simulink model "test_control_lib_vect_sign_change"  (R2017a)
settings: Solver=VariableStepAuto  StartTime=0.0  StopTime=0.020*100  RelTol=1e-3
settings Model: Creator=CHIVFUR  LastModifiedBy=CHIVFUR

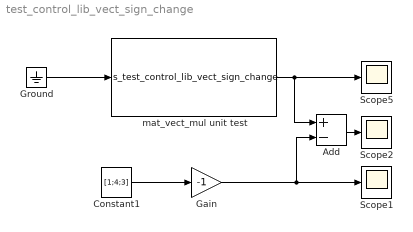
== system test_control_lib_vect_sign_change ==
  Add : Sum  Inputs=+-
  Constant1 : Constant  Value=[1;4;3]
  Gain : Gain  Gain=-1
  Ground : Ground
  Scope1 : Scope
  Scope2 : Scope
  Scope5 : Scope
  "mat_vect_mul unit test " : S-Function  FunctionName=s_test_control_lib_vect_sign_change  Parameters=1/30000  SFunctionDeploymentMode=off  EnableBusSupport=off
  wires:
  "mat_vect_mul unit test "/1 -> Scope5/1, Add/1
  Ground/1 -> "mat_vect_mul unit test "/1
  Constant1/1 -> Gain/1
  Add/1 -> Scope2/1
  Gain/1 -> Scope1/1, Add/2
